simulink model "Ieee14"  (R2023b)
settings: Solver=ode1  StartTime=0.0  StopTime=600  FixedStep=1e-3  MaxStep=1e-4  RelTol=1e-3
model workspace (MAT data in the model file):
  pruebaValor = 0
undefined symbols (not defined in the file or in its folder): f
libraries: spsThreePhaseVIMeasurementLib x39, spsThreePhaseBreakerLib x21, spsLoadFlowBusLib x19, spsThreePhaseSeriesRLCBranchLib x16, spsThreePhaseFaultLib x16, source_mod x14, instrumentlib x8, spsThreePhaseTransformerTwoWindingsLib x4, spsThreePhaseSourceLib x2, spspowerguiLib x1
(part 2 of 2)

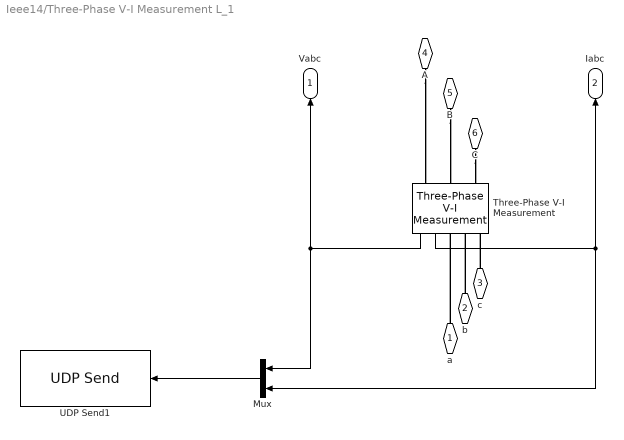
== system Ieee14/Three-Phase V-I Measurement L_1 ==
  Mux : Mux  Inputs=2
  Three-Phase V-I Measurement : spsThreePhaseVIMeasurementLib/Three-Phase V-I Measurement  VoltageMeasurement=phase-to-ground  SetLabelV=off  LabelV=Vabc  Vpu=off  VpuLL=off  CurrentMeasurement=yes  SetLabelI=off  LabelI=Iabc  Ipu=off  Pbase=1e3  Vbase=13.8e3  OutputType=Complex  PhasorSimulation=off  PSBequivalent=0
  UDP Send1 : instrumentlib/UDP Send  Host=10.0.1.1  Port=10001  LocalAddress=0.0.0.0  LocalPort=-1  EnablePortSharing=off  OutputDatagramPacketSize=512  ByteOrder=big-endian  EnableBlockingMode=on  SimulateUsing=Interpreted execution
  a : PMIOPort  Side=Left
  b : PMIOPort  Port=2  Side=Left
  c : PMIOPort  Port=3  Side=Left
  A : PMIOPort  Port=4  Side=Right
  B : PMIOPort  Port=5  Side=Right
  C : PMIOPort  Port=6  Side=Right
  Vabc : Outport
  Iabc : Outport  Port=2
  wires:
  Three-Phase V-I Measurement/1 -> Vabc/1, Mux/1
  Three-Phase V-I Measurement/2 -> Mux/2, Iabc/1
  Mux/1 -> UDP Send1/1
  connections:
  b/RConn1 -- Three-Phase V-I Measurement/RConn2
  a/RConn1 -- Three-Phase V-I Measurement/RConn1
  c/RConn1 -- Three-Phase V-I Measurement/RConn3
  A/RConn1 -- Three-Phase V-I Measurement/LConn1
  B/RConn1 -- Three-Phase V-I Measurement/LConn2
  C/RConn1 -- Three-Phase V-I Measurement/LConn3

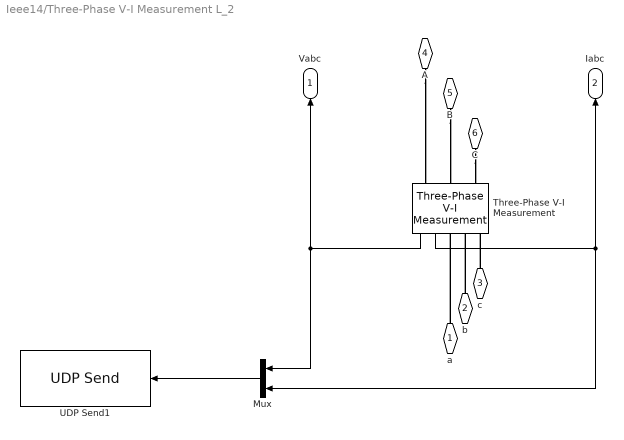
== system Ieee14/Three-Phase V-I Measurement L_2 ==
  Mux : Mux  Inputs=2
  Three-Phase V-I Measurement : spsThreePhaseVIMeasurementLib/Three-Phase V-I Measurement  VoltageMeasurement=phase-to-ground  SetLabelV=off  LabelV=Vabc  Vpu=off  VpuLL=off  CurrentMeasurement=yes  SetLabelI=off  LabelI=Iabc  Ipu=off  Pbase=1e3  Vbase=13.8e3  OutputType=Complex  PhasorSimulation=off  PSBequivalent=0
  UDP Send1 : instrumentlib/UDP Send  Host=10.0.2.1  Port=10002  LocalAddress=0.0.0.0  LocalPort=-1  EnablePortSharing=off  OutputDatagramPacketSize=512  ByteOrder=big-endian  EnableBlockingMode=on  SimulateUsing=Interpreted execution
  a : PMIOPort  Side=Left
  b : PMIOPort  Port=2  Side=Left
  c : PMIOPort  Port=3  Side=Left
  A : PMIOPort  Port=4  Side=Right
  B : PMIOPort  Port=5  Side=Right
  C : PMIOPort  Port=6  Side=Right
  Vabc : Outport
  Iabc : Outport  Port=2
  wires:
  Three-Phase V-I Measurement/1 -> Vabc/1, Mux/1
  Three-Phase V-I Measurement/2 -> Mux/2, Iabc/1
  Mux/1 -> UDP Send1/1
  connections:
  b/RConn1 -- Three-Phase V-I Measurement/RConn2
  a/RConn1 -- Three-Phase V-I Measurement/RConn1
  c/RConn1 -- Three-Phase V-I Measurement/RConn3
  A/RConn1 -- Three-Phase V-I Measurement/LConn1
  B/RConn1 -- Three-Phase V-I Measurement/LConn2
  C/RConn1 -- Three-Phase V-I Measurement/LConn3

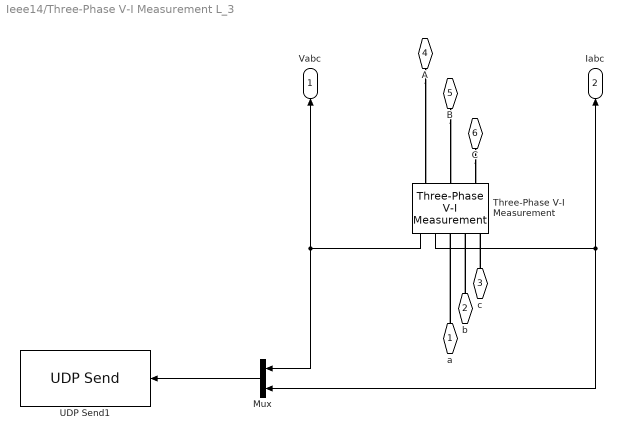
== system Ieee14/Three-Phase V-I Measurement L_3  ==
  Mux : Mux  Inputs=2
  Three-Phase V-I Measurement : spsThreePhaseVIMeasurementLib/Three-Phase V-I Measurement  VoltageMeasurement=phase-to-ground  SetLabelV=off  LabelV=Vabc  Vpu=off  VpuLL=off  CurrentMeasurement=yes  SetLabelI=off  LabelI=Iabc  Ipu=off  Pbase=1e3  Vbase=13.8e3  OutputType=Complex  PhasorSimulation=off  PSBequivalent=0
  UDP Send1 : instrumentlib/UDP Send  Host=10.0.3.1  Port=10003  LocalAddress=0.0.0.0  LocalPort=-1  EnablePortSharing=off  OutputDatagramPacketSize=512  ByteOrder=big-endian  EnableBlockingMode=on  SimulateUsing=Interpreted execution
  a : PMIOPort  Side=Left
  b : PMIOPort  Port=2  Side=Left
  c : PMIOPort  Port=3  Side=Left
  A : PMIOPort  Port=4  Side=Right
  B : PMIOPort  Port=5  Side=Right
  C : PMIOPort  Port=6  Side=Right
  Vabc : Outport
  Iabc : Outport  Port=2
  wires:
  Three-Phase V-I Measurement/1 -> Vabc/1, Mux/1
  Three-Phase V-I Measurement/2 -> Mux/2, Iabc/1
  Mux/1 -> UDP Send1/1
  connections:
  b/RConn1 -- Three-Phase V-I Measurement/RConn2
  a/RConn1 -- Three-Phase V-I Measurement/RConn1
  c/RConn1 -- Three-Phase V-I Measurement/RConn3
  A/RConn1 -- Three-Phase V-I Measurement/LConn1
  B/RConn1 -- Three-Phase V-I Measurement/LConn2
  C/RConn1 -- Three-Phase V-I Measurement/LConn3

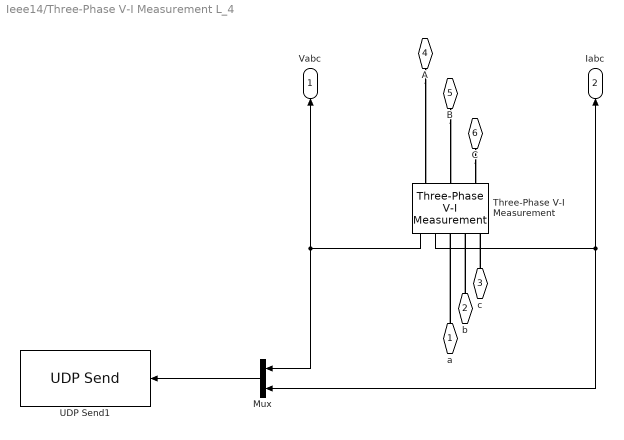
== system Ieee14/Three-Phase V-I Measurement L_4 ==
  Mux : Mux  Inputs=2
  Three-Phase V-I Measurement : spsThreePhaseVIMeasurementLib/Three-Phase V-I Measurement  VoltageMeasurement=phase-to-ground  SetLabelV=off  LabelV=Vabc  Vpu=off  VpuLL=off  CurrentMeasurement=yes  SetLabelI=off  LabelI=Iabc  Ipu=off  Pbase=1e3  Vbase=13.8e3  OutputType=Complex  PhasorSimulation=off  PSBequivalent=0
  UDP Send1 : instrumentlib/UDP Send  Host=10.0.4.1  Port=10004  LocalAddress=0.0.0.0  LocalPort=-1  EnablePortSharing=off  OutputDatagramPacketSize=512  ByteOrder=big-endian  EnableBlockingMode=on  SimulateUsing=Interpreted execution
  a : PMIOPort  Side=Left
  b : PMIOPort  Port=2  Side=Left
  c : PMIOPort  Port=3  Side=Left
  A : PMIOPort  Port=4  Side=Right
  B : PMIOPort  Port=5  Side=Right
  C : PMIOPort  Port=6  Side=Right
  Vabc : Outport
  Iabc : Outport  Port=2
  wires:
  Three-Phase V-I Measurement/1 -> Vabc/1, Mux/1
  Three-Phase V-I Measurement/2 -> Mux/2, Iabc/1
  Mux/1 -> UDP Send1/1
  connections:
  b/RConn1 -- Three-Phase V-I Measurement/RConn2
  a/RConn1 -- Three-Phase V-I Measurement/RConn1
  c/RConn1 -- Three-Phase V-I Measurement/RConn3
  A/RConn1 -- Three-Phase V-I Measurement/LConn1
  B/RConn1 -- Three-Phase V-I Measurement/LConn2
  C/RConn1 -- Three-Phase V-I Measurement/LConn3

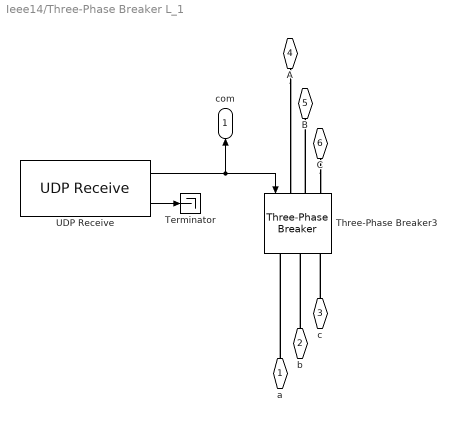
== system Ieee14/Three-Phase Breaker L_1 ==
  Terminator : Terminator
  Three-Phase Breaker3 : spsThreePhaseBreakerLib/Three-Phase Breaker  InitialState=closed  SwitchA=on  SwitchB=on  SwitchC=on  SwitchTimes=[0.2]  External=on  BreakerResistance=0.01  SnubberResistance=1e6  SnubberCapacitance=inf  Measurements=Breaker voltages and currents
  UDP Receive : instrumentlib/UDP Receive  LocalAddress=0.0.0.0  LocalPort=20001  EnablePortSharing=off  Host=10.0.1.2  Port=20001  GetLatestData=off  DataSize=[ 1, 1 ]  DataType=uint16  ASCIIFormatting=%f,  Terminator=LF  CustomTerminator=10  ByteOrder=big-endian  EnableBlockingMode=off  Timeout=10  SampleTime=0.01  SimulateUsing=Interpreted execution
  a : PMIOPort  Side=Left
  b : PMIOPort  Port=2  Side=Left
  c : PMIOPort  Port=3  Side=Left
  A : PMIOPort  Port=4  Side=Right
  B : PMIOPort  Port=5  Side=Right
  C : PMIOPort  Port=6  Side=Right
  com : Outport
  wires:
  UDP Receive/1 -> com/1, Three-Phase Breaker3/1
  UDP Receive/2 -> Terminator/1
  connections:
  b/RConn1 -- Three-Phase Breaker3/RConn2
  c/RConn1 -- Three-Phase Breaker3/RConn3
  A/RConn1 -- Three-Phase Breaker3/LConn1
  Three-Phase Breaker3/LConn2 -- B/RConn1
  C/RConn1 -- Three-Phase Breaker3/LConn3
  a/RConn1 -- Three-Phase Breaker3/RConn1

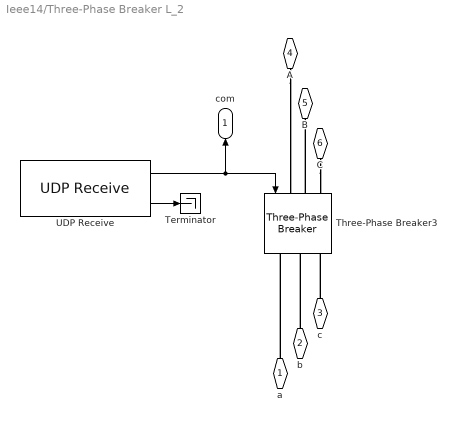
== system Ieee14/Three-Phase Breaker L_2 ==
  Terminator : Terminator
  Three-Phase Breaker3 : spsThreePhaseBreakerLib/Three-Phase Breaker  InitialState=closed  SwitchA=on  SwitchB=on  SwitchC=on  SwitchTimes=[0.2]  External=on  BreakerResistance=0.01  SnubberResistance=1e6  SnubberCapacitance=inf  Measurements=Breaker voltages and currents
  UDP Receive : instrumentlib/UDP Receive  LocalAddress=0.0.0.0  LocalPort=20002  EnablePortSharing=off  Host=10.0.2.2  Port=20002  GetLatestData=off  DataSize=[ 1, 1 ]  DataType=uint16  ASCIIFormatting=%f,  Terminator=LF  CustomTerminator=10  ByteOrder=big-endian  EnableBlockingMode=off  Timeout=10  SampleTime=0.01  SimulateUsing=Interpreted execution
  a : PMIOPort  Side=Left
  b : PMIOPort  Port=2  Side=Left
  c : PMIOPort  Port=3  Side=Left
  A : PMIOPort  Port=4  Side=Right
  B : PMIOPort  Port=5  Side=Right
  C : PMIOPort  Port=6  Side=Right
  com : Outport
  wires:
  UDP Receive/1 -> com/1, Three-Phase Breaker3/1
  UDP Receive/2 -> Terminator/1
  connections:
  b/RConn1 -- Three-Phase Breaker3/RConn2
  c/RConn1 -- Three-Phase Breaker3/RConn3
  A/RConn1 -- Three-Phase Breaker3/LConn1
  Three-Phase Breaker3/LConn2 -- B/RConn1
  C/RConn1 -- Three-Phase Breaker3/LConn3
  a/RConn1 -- Three-Phase Breaker3/RConn1

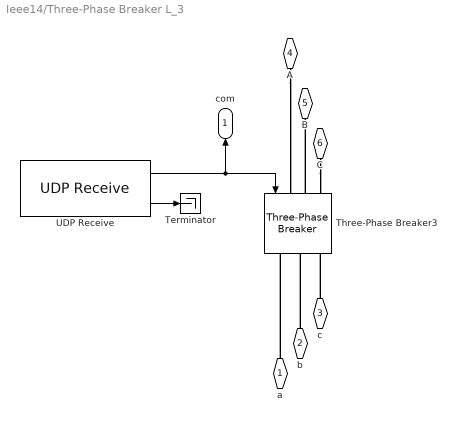
== system Ieee14/Three-Phase Breaker L_3 ==
  Terminator : Terminator
  Three-Phase Breaker3 : spsThreePhaseBreakerLib/Three-Phase Breaker  InitialState=closed  SwitchA=on  SwitchB=on  SwitchC=on  SwitchTimes=[0.2]  External=on  BreakerResistance=0.01  SnubberResistance=1e6  SnubberCapacitance=inf  Measurements=Breaker voltages and currents
  UDP Receive : instrumentlib/UDP Receive  LocalAddress=0.0.0.0  LocalPort=20003  EnablePortSharing=off  Host=10.0.3.2  Port=20003  GetLatestData=off  DataSize=[ 1, 1 ]  DataType=uint16  ASCIIFormatting=%f,  Terminator=LF  CustomTerminator=10  ByteOrder=big-endian  EnableBlockingMode=off  Timeout=10  SampleTime=0.01  SimulateUsing=Interpreted execution
  a : PMIOPort  Side=Left
  b : PMIOPort  Port=2  Side=Left
  c : PMIOPort  Port=3  Side=Left
  A : PMIOPort  Port=4  Side=Right
  B : PMIOPort  Port=5  Side=Right
  C : PMIOPort  Port=6  Side=Right
  com : Outport
  wires:
  UDP Receive/1 -> com/1, Three-Phase Breaker3/1
  UDP Receive/2 -> Terminator/1
  connections:
  b/RConn1 -- Three-Phase Breaker3/RConn2
  c/RConn1 -- Three-Phase Breaker3/RConn3
  A/RConn1 -- Three-Phase Breaker3/LConn1
  Three-Phase Breaker3/LConn2 -- B/RConn1
  C/RConn1 -- Three-Phase Breaker3/LConn3
  a/RConn1 -- Three-Phase Breaker3/RConn1

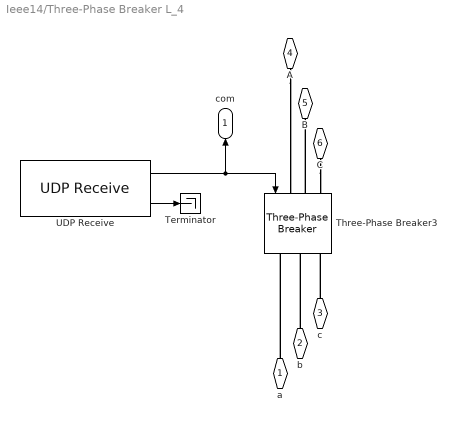
== system Ieee14/Three-Phase Breaker L_4 ==
  Terminator : Terminator
  Three-Phase Breaker3 : spsThreePhaseBreakerLib/Three-Phase Breaker  InitialState=closed  SwitchA=on  SwitchB=on  SwitchC=on  SwitchTimes=[0.2]  External=on  BreakerResistance=0.01  SnubberResistance=1e6  SnubberCapacitance=inf  Measurements=Breaker voltages and currents
  UDP Receive : instrumentlib/UDP Receive  LocalAddress=0.0.0.0  LocalPort=20004  EnablePortSharing=off  Host=10.0.4.2  Port=20004  GetLatestData=off  DataSize=[ 1, 1 ]  DataType=uint16  ASCIIFormatting=%f,  Terminator=LF  CustomTerminator=10  ByteOrder=big-endian  EnableBlockingMode=off  Timeout=10  SampleTime=0.01  SimulateUsing=Interpreted execution
  a : PMIOPort  Side=Left
  b : PMIOPort  Port=2  Side=Left
  c : PMIOPort  Port=3  Side=Left
  A : PMIOPort  Port=4  Side=Right
  B : PMIOPort  Port=5  Side=Right
  C : PMIOPort  Port=6  Side=Right
  com : Outport
  wires:
  UDP Receive/1 -> com/1, Three-Phase Breaker3/1
  UDP Receive/2 -> Terminator/1
  connections:
  b/RConn1 -- Three-Phase Breaker3/RConn2
  c/RConn1 -- Three-Phase Breaker3/RConn3
  A/RConn1 -- Three-Phase Breaker3/LConn1
  Three-Phase Breaker3/LConn2 -- B/RConn1
  C/RConn1 -- Three-Phase Breaker3/LConn3
  a/RConn1 -- Three-Phase Breaker3/RConn1

== matlab function Ieee14/startFcn ==
  settings: sampleTime=0
  data: u input
function fcn(u)

%{

Function: startFcn

Details: Initialization function for the network. It runs only once. 
Calls the external resetRed function, which initializes the network's values.

Additional: To suppress any warning messages, they are disabled with the line 
warning('off','all'). Despite the warning, it does not affect the network's functionality.

%}


% - - - - - - - - - - - - - - - - - - - - - - - - -

% Coder
coder.extrinsic('resetRed');
coder.extrinsic('warning');

% - - - - - - - - - - - - - - - - - - - - - - - - -

% Reset
if u == 0
    resetRed();
    warning('off','all');
end

% - - - - - - - - - - - - - - - - - - - - - - - - -
end

== matlab function Ieee14/SC ==
  settings: updateMethod=DISCRETE  sampleTime=20
function fcn()

    %{
    
    Function SC: short circuits (faults).
    
    Details: This function is responsible for causing short circuits
    throughout the simulation.
    
    Important: In the "edit Data" section, you must adjust the time interval 
    for entering this function. If the value is set to 20 seconds, its behavior is: 
    
    T = 5s   --> SC is activated
    T = 10s  --> SC is deactivated
    T = 15s  --> SC is activated
    T = 20s  --> SC is deactivated
    ... ... ...
    
    %}
    
    % - - - - - - - - - - - - - - - - - - - - - - - - -
    
    % coders
    coder.extrinsic('mat2str');
    coder.extrinsic('set_param');
    
    % - - - - - - - - - - - - - - - - - - - - - - - - -
    
    % Variable settings
    % If "jump" is 1, SC will not be activated. Set it to 0. 
    jump = 0;
    
    % - - - - - - - - - - - - - - - - - - - - - - - - -
    
    % = = = = = = = = = = = = = = = = = = = = = = = = =
    % = = = = = = = = = = = = = = = = = = = = = = = = =
    % - - - - - - - - -  Code - - - - - - - - - - - - - 
    % = = = = = = = = = = = = = = = = = = = = = = = = =
    % = = = = = = = = = = = = = = = = = = = = = = = = =
    
    % - - - - - - - - - - - - - - - - - - - - - - - - -
    
    % Activate or desativate function
    if jump == 1
        return
    end
    
    % - - - - - - - - - - - - - - - - - - - - - - - - -
    
    % Persistent variables
    
    % attack: if it is 1, the short circuit (SC) occurs
    persistent attack
    if isempty(attack)
       attack = 0;
       return
    end
    
    % lineSC: line that has a short circuit
    persistent lineSC;
    if isempty(lineSC)
        lineSC = 0;
    end
    
    % - - - - - - - - - - - - - - - - - - - - - - - - -
    
    % Model address
    address = "Ieee14/";
    
    % - - - - - - - - - - - - - - - - - - - - - - - - -
    
    % Restore attack
    if attack == 1
        if lineSC == 1
            line = "L1";
            aux = address + "SC_" + line;
            set_param(aux, 'Value', mat2str(0));
        end
        if lineSC == 2
            line = "L2";
            aux = address + "SC_" + line;
            set_param(aux, 'Value', mat2str(0));
        end
        if lineSC == 3
            line = "L3";
            aux = address + "SC_" + line;
            set_param(aux, 'Value', mat2str(0));
        end
        if lineSC == 4
            line = "L4";
            aux = address + "SC_" + line;
            set_param(aux, 'Value', mat2str(0));
        end
        if lineSC == 5
            line = "B2_L4";
            aux = address + "SC_" + line;
            set_param(aux, 'Value', mat2str(0));
        end
        if lineSC == 6
            line = "B2_G3";
            aux = address + "SC_" + line;
            set_param(aux, 'Value', mat2str(0));
        end
        if lineSC == 7
            line = "B3_L4";
            aux = address + "SC_" + line;
            set_param(aux, 'Value', mat2str(0));
        end
        if lineSC == 8
            line = "B1_L5";
            aux = address + "SC_" + line;
            set_param(aux, 'Value', mat2str(0));
        end
        if lineSC == 9
            line = "B1_L4";
            aux = address + "SC_" + line;
            set_param(aux, 'Value', mat2str(0));
        end
        if lineSC == 10
            line = "B2_G1";
            aux = address + "SC_" + line;
            set_param(aux, 'Value', mat2str(0));
        end
        if lineSC == 11
            line = "B2_L5";
            aux = address + "SC_" + line;
            set_param(aux, 'Value', mat2str(0));
        end
        if lineSC == 12
            line = "B6_L10";
            aux = address + "SC_" + line;
            set_param(aux, 'Value', mat2str(0));
        end
        if lineSC == 13
            line = "B6_L14";
            aux = address + "SC_" + line;
            set_param(aux, 'Value', mat2str(0));
        end
        if lineSC == 14
            line = "B8_L5";
            aux = address + "SC_" + line;
            set_param(aux, 'Value', mat2str(0));
        end
        if lineSC == 15
            line = "B8_L14";
            aux = address + "SC_" + line;
            set_param(aux, 'Value', mat2str(0));
        end
        if lineSC == 16
            line = "B8_L10";
            aux = address + "SC_" + line;
            set_param(aux, 'Value', mat2str(0));
        end
    
        attack = 0;
        disp('=============')
        disp('Disconnection of SC');
        disp('=============');
        return
    end
    
    % Activate short circuit
    
    if attack == 0
        lineSC = randi(16);
        disp('=======================');
        disp('=======================');
        disp('lineSC');
        disp(lineSC);
        disp('=======================');
        disp('=======================');
        if lineSC == 1
            line = "L1";
            aux = address + "SC_" + line;
            set_param(aux, 'Value', mat2str(1));
        end
        if lineSC == 2
            line = "L2";
            aux = address + "SC_" + line;
            set_param(aux, 'Value', mat2str(1));
        end
        if lineSC == 3
            line = "L3";
            aux = address + "SC_" + line;
            set_param(aux, 'Value', mat2str(1));
        end
        if lineSC == 4
            line = "L4";
            aux = address + "SC_" + line;
            set_param(aux, 'Value', mat2str(1));
        end
        if lineSC == 5
            line = "B2_L4";
            aux = address + "SC_" + line;
            set_param(aux, 'Value', mat2str(1));
        end
        if lineSC == 6
            line = "B2_G3";
            aux = address + "SC_" + line;
            set_param(aux, 'Value', mat2str(1));
        end
        if lineSC == 7
            line = "B3_L4";
            aux = address + "SC_" + line;
            set_param(aux, 'Value', mat2str(1));
        end
        if lineSC == 8
            line = "B1_L5";
            aux = address + "SC_" + line;
            set_param(aux, 'Value', mat2str(1));
        end
        if lineSC == 9
            line = "B1_L4";
            aux = address + "SC_" + line;
            set_param(aux, 'Value', mat2str(1));
        end
        if lineSC == 10
            line = "B2_G1";
            aux = address + "SC_" + line;
            set_param(aux, 'Value', mat2str(1));
        end
        if lineSC == 11
            line = "B2_L5";
            aux = address + "SC_" + line;
            set_param(aux, 'Value', mat2str(1));
        end
        if lineSC == 12
            line = "B6_L10";
            aux = address + "SC_" + line;
            set_param(aux, 'Value', mat2str(1));
        end
        if lineSC == 13
            line = "B6_L14";
            aux = address + "SC_" + line;
            set_param(aux, 'Value', mat2str(1));
        end
        if lineSC == 14
            line = "B8_L5";
            aux = address + "SC_" + line;
            set_param(aux, 'Value', mat2str(1));
        end
        if lineSC == 15
            line = "B8_L14";
            aux = address + "SC_" + line;
            set_param(aux, 'Value', mat2str(1));
        end
        if lineSC == 16
            line = "B8_L10";
            aux = address + "SC_" + line;
            set_param(aux, 'Value', mat2str(1));
        end
        attack = 1;
        return
    end

end
